simulink model "sixdof"  (R2023a)
settings: Solver=FixedStepAuto  StartTime=0.0  StopTime=5000  FixedStep=0.01  RelTol=1e-3  EnableMultiTasking=on
InitFcn:
  | fox_loadvariables_new
model workspace (MAT data in the model file):
  waypoints = [0 1000 1000 -1000 0 0 0 1000 1000 0 20 20 ... (15 elements, 5x3)]
values from neighbouring files (symbols this model uses):
  Apolar = 0.038    [fox_loadvariables_new.m]
  CD0 = 0.0191    [fox_loadvariables_new.m]
  chord = chord*0.3048    (= 0.3048)    [fox_loadvariables_new.m]
  CL0 = 3*0.076    (= 0.228)    [fox_loadvariables_new.m]
  CLa = 5.097    [fox_loadvariables_new.m]
  CLa_dot = 1.93    [fox_loadvariables_new.m]
  Clb = -0.0598    [fox_loadvariables_new.m]
  ClDa = 0.265    [fox_loadvariables_new.m]
  CLDe = 0.738    [fox_loadvariables_new.m]
  ClDr = 0.0064    [fox_loadvariables_new.m]
  Clp = -0.363    [fox_loadvariables_new.m]
  CLq = 6.03    [fox_loadvariables_new.m]
  Clr = 0.0886    [fox_loadvariables_new.m]
  Cm0 = 0.107    [fox_loadvariables_new.m]
  Cma = -2.051    [fox_loadvariables_new.m]
  Cma_dot = -5.286    [fox_loadvariables_new.m]
  CmDe = -2.021    [fox_loadvariables_new.m]
  Cmq = -16.52    [fox_loadvariables_new.m]
  Cnb = 0.0562    [fox_loadvariables_new.m]
  CnDa = -0.0296    [fox_loadvariables_new.m]
  CnDr = -0.0377    [fox_loadvariables_new.m]
  Cnp = -0.0407    [fox_loadvariables_new.m]
  Cnr = -0.0439    [fox_loadvariables_new.m]
  CYb = -0.204    [fox_loadvariables_new.m]
  CYDr = 0.112    [fox_loadvariables_new.m]
  Euler_0 = [0; 0; 180]'*pi/180    [fox_loadvariables_new.m]
  ISA_g = 9.815    [fox_loadvariables_new.m]
  ISA_hmax = 2000    [fox_loadvariables_new.m]
  ISA_lapse = .0065    (= 0.0065)    [fox_loadvariables_new.m]
  ISA_P0 = 101325    [fox_loadvariables_new.m]
  ISA_R = 287    [fox_loadvariables_new.m]
  ISA_rho0 = 1.225    [fox_loadvariables_new.m]
  ISA_T0 = 289    [fox_loadvariables_new.m]
  Ixx = Ixx*1.355817949    (= 0.363359210332)    [fox_loadvariables_new.m]
  Iyy = Iyy*1.355817949    (= 0.86772348736)    [fox_loadvariables_new.m]
  Izz = Izz*1.355817949    (= 1.19854306692)    [fox_loadvariables_new.m]
  mass = mass*0.45359237    (= 9.0718474)    [fox_loadvariables_new.m]
  Pos_0 = [0; 0; 100.]    [fox_loadvariables_new.m]
  PQR_0 = [0; 0; 0]'    [fox_loadvariables_new.m]
  span = span*0.3048    (= 2.4384)    [fox_loadvariables_new.m]
  Vb_0 = [85.; 0; 0]'*0.3048    [fox_loadvariables_new.m]
undefined symbols (not defined in the file or in its folder): YPGwind
libraries: simulink x5, slpidlib x5, sharedtransform x1, uavutilslib x1, uavalgslib x1
(part 2 of 2)

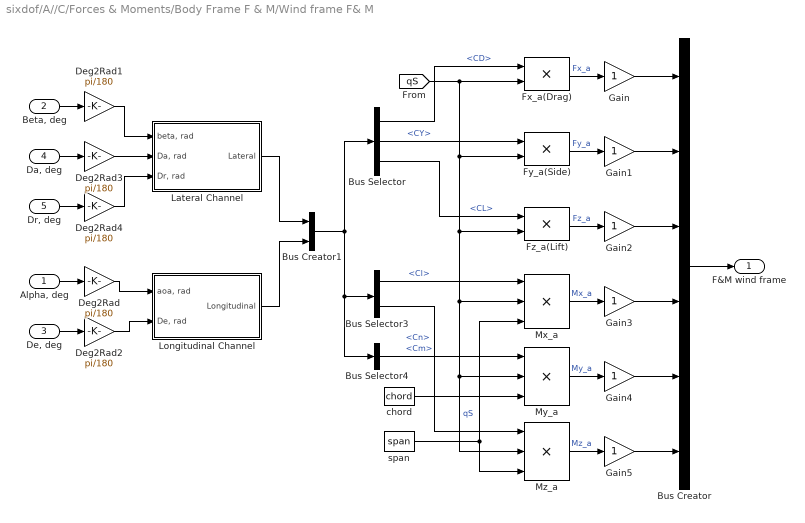
== system sixdof/A//C/Forces & Moments/Body Frame F & M/Wind frame F& M ==
  "Alpha, deg" : Inport
  "Beta, deg" : Inport  Port=2
  "De, deg" : Inport  Port=3
  "Da, deg" : Inport  Port=4
  "Dr, deg" : Inport  Port=5
  Bus Creator : BusCreator  Inputs=6
  Bus Creator1 : BusCreator  Inputs=2
  Bus Selector : BusSelector  OutputSignals=signal2.CD,signal1.CY,signal2.CL
  Bus Selector3 : BusSelector  OutputSignals=signal1.Cl,signal1.Cn
  Bus Selector4 : BusSelector  OutputSignals=signal2.Cm
  Deg2Rad{,1..4} (5 alike) : Gain  Gain=pi/180  SaturateOnIntegerOverflow=on  OutDataTypeStr=Inherit: Same as input  ParamDataTypeStr=Inherit: Same as input
  Fx_a(Drag) : Product  Inputs=**  SaturateOnIntegerOverflow=on  OutDataTypeStr=Inherit: Same as first input
  Fy_a(Side) : Product  SaturateOnIntegerOverflow=on  OutDataTypeStr=Inherit: Same as first input
  Fz_a(Lift) : Product  SaturateOnIntegerOverflow=on  OutDataTypeStr=Inherit: Same as first input
  Gain{,1..5} (6 alike) : Gain  SaturateOnIntegerOverflow=on  OutDataTypeStr=Inherit: Same as input  ParamDataTypeStr=Inherit: Same as input
  Lateral Channel : Subsystem
  Longitudinal Channel : Subsystem
  Mx_a : Product  Inputs=3  SaturateOnIntegerOverflow=on  OutDataTypeStr=Inherit: Same as first input
  My_a : Product  Inputs=3  SaturateOnIntegerOverflow=on  OutDataTypeStr=Inherit: Same as first input
  Mz_a : Product  Inputs=3  SaturateOnIntegerOverflow=on  OutDataTypeStr=Inherit: Same as first input
  chord : Constant  Value=chord  VectorParams1D=off
  span : Constant  Value=span  VectorParams1D=off
  F&M wind frame : Outport
  wires:
  Bus Selector/1 -> Fx_a(Drag)/1  "<CD>"
  Fx_a(Drag)/1 -> Gain/1  "Fx_a"
  Fy_a(Side)/1 -> Gain1/1  "Fy_a"
  Fz_a(Lift)/1 -> Gain2/1  "Fz_a"
  Bus Selector3/1 -> Mx_a/1  "<Cl>"
  Mx_a/1 -> Gain3/1  "Mx_a"
  Bus Selector4/1 -> My_a/1  "<Cm>"
  Mz_a/1 -> Gain5/1  "Mz_a"
  [qS] -> Fx_a(Drag)/2, Fy_a(Side)/2, Fz_a(Lift)/2, Mx_a/2, My_a/2, Mz_a/2  "qS"
  span/1 -> Mx_a/3, Mz_a/3
  chord/1 -> My_a/3
  Bus Selector/2 -> Fy_a(Side)/1  "<CY>"
  Bus Selector/3 -> Fz_a(Lift)/1  "<CL>"
  Bus Selector3/2 -> Mz_a/1  "<Cn>"
  Bus Creator/1 -> F&M wind frame/1
  My_a/1 -> Gain4/1  "My_a"
  Bus Creator1/1 -> Bus Selector/1, Bus Selector3/1, Bus Selector4/1
  Lateral Channel/1(Lateral) -> Bus Creator1/1
  Longitudinal Channel/1(Longitudinal) -> Bus Creator1/2
  "Alpha, deg"/1 -> Deg2Rad/1
  "Beta, deg"/1 -> Deg2Rad1/1
  "De, deg"/1 -> Deg2Rad2/1
  "Da, deg"/1 -> Deg2Rad3/1
  "Dr, deg"/1 -> Deg2Rad4/1
  Deg2Rad1/1 -> Lateral Channel/1("beta, rad")
  Deg2Rad3/1 -> Lateral Channel/2("Da, rad")
  Deg2Rad4/1 -> Lateral Channel/3("Dr, rad")
  Deg2Rad/1 -> Longitudinal Channel/1("aoa, rad")
  Deg2Rad2/1 -> Longitudinal Channel/2("De, rad")
  Gain/1 -> Bus Creator/1
  Gain1/1 -> Bus Creator/2
  Gain2/1 -> Bus Creator/3
  Gain3/1 -> Bus Creator/4
  Gain4/1 -> Bus Creator/5
  Gain5/1 -> Bus Creator/6

== system sixdof/A//C/Forces & Moments/U2B1/Rb2u ==
  phi theta psi : Inport
  11 : Fcn  Expr=cos(u[3])*cos(u[2])
  12 : Fcn  Expr=sin(u[3])*cos(u[2])
  13 : Fcn  Expr=-sin(u[2])
  21 : Fcn  Expr=cos(u[3])*sin(u[2])*sin(u[1])-sin(u[3])*cos(u[1])
  22 : Fcn  Expr=sin(u[3])*sin(u[2])*sin(u[1])+cos(u[3])*cos(u[1])
  23 : Fcn  Expr=cos(u[2])*sin(u[1])
  31 : Fcn  Expr=cos(u[3])*sin(u[2])*cos(u[1])+sin(u[3])*sin(u[1])
  32 : Fcn  Expr=sin(u[3])*sin(u[2])*cos(u[1])-cos(u[3])*sin(u[1])
  33 : Fcn  Expr=cos(u[2])*cos(u[1])
  Mux2 : Mux  Inputs=9
  Reshape : Reshape  OutputDimensionality=Customize  OutputDimensions=[3,3]
  DCM : Outport  InitialOutput=0
  wires:
  Reshape/1 -> DCM/1
  phi theta psi/1 -> 12/1, 13/1, 21/1, 22/1, 23/1, 31/1, 32/1, 33/1, 11/1
  Mux2/1 -> Reshape/1
  11/1 -> Mux2/1
  12/1 -> Mux2/2
  13/1 -> Mux2/3
  21/1 -> Mux2/4
  22/1 -> Mux2/5
  23/1 -> Mux2/6
  31/1 -> Mux2/7
  32/1 -> Mux2/8
  33/1 -> Mux2/9

== system sixdof/A//C/Forces & Moments/U2B2/Rb2u ==
  phi theta psi : Inport
  11 : Fcn  Expr=cos(u[3])*cos(u[2])
  12 : Fcn  Expr=sin(u[3])*cos(u[2])
  13 : Fcn  Expr=-sin(u[2])
  21 : Fcn  Expr=cos(u[3])*sin(u[2])*sin(u[1])-sin(u[3])*cos(u[1])
  22 : Fcn  Expr=sin(u[3])*sin(u[2])*sin(u[1])+cos(u[3])*cos(u[1])
  23 : Fcn  Expr=cos(u[2])*sin(u[1])
  31 : Fcn  Expr=cos(u[3])*sin(u[2])*cos(u[1])+sin(u[3])*sin(u[1])
  32 : Fcn  Expr=sin(u[3])*sin(u[2])*cos(u[1])-cos(u[3])*sin(u[1])
  33 : Fcn  Expr=cos(u[2])*cos(u[1])
  Mux2 : Mux  Inputs=9
  Reshape : Reshape  OutputDimensionality=Customize  OutputDimensions=[3,3]
  DCM : Outport  InitialOutput=0
  wires:
  33/1 -> Mux2/9
  32/1 -> Mux2/8
  31/1 -> Mux2/7
  23/1 -> Mux2/6
  22/1 -> Mux2/5
  21/1 -> Mux2/4
  13/1 -> Mux2/3
  12/1 -> Mux2/2
  11/1 -> Mux2/1
  Mux2/1 -> Reshape/1
  phi theta psi/1 -> 11/1, 33/1, 32/1, 31/1, 23/1, 22/1, 21/1, 13/1, 12/1
  Reshape/1 -> DCM/1

== system sixdof/A//C/ISA Atmosphere & Winds/Wind model/GetWind ==
  Alt : Inport
  "   " : Gain  SaturateOnIntegerOverflow=on  OutDataTypeStr=Inherit: Same as input  ParamDataTypeStr=Inherit: Same as input
  "   1" : Gain  SaturateOnIntegerOverflow=on  OutDataTypeStr=Inherit: Same as input  ParamDataTypeStr=Inherit: Same as input
  "   2" : Gain  SaturateOnIntegerOverflow=on  OutDataTypeStr=Inherit: Same as input  ParamDataTypeStr=Inherit: Same as input
  Mux : Mux  Inputs=3
  WindX : Lookup  InputValues=YPGwind(:,1)  Table=YPGwind(:,3)
  WindY : Lookup  InputValues=YPGwind(:,1)  Table=YPGwind(:,2)
  WindZ : Lookup  InputValues=YPGwind(:,1)  Table=YPGwind(:,4)
  WindOut : Outport  InitialOutput=0
  wires:
  WindY/1 -> "   1"/1
  Alt/1 -> WindZ/1, WindX/1, WindY/1
  WindX/1 -> "   "/1
  "   1"/1 -> Mux/2
  "   "/1 -> Mux/1
  "   2"/1 -> Mux/3
  WindZ/1 -> "   2"/1
  Mux/1 -> WindOut/1

== system sixdof/A//C/Forces & Moments/Body Frame F & M/Transfer to body frame/Ra2b1 ==
  wind frame : Inport
  aoa/beta : Inport  Port=2
  Product2 : Product  Multiplication=Matrix(*)  SaturateOnIntegerOverflow=on  OutDataTypeStr=Inherit: Same as first input
  Ra2b : Math  Operator=transpose  SignedPower=on
  Rb2a : Subsystem
  Reshape : Reshape  OutputDimensionality=Column vector (2-D)
  body frame : Outport
  wires:
  Rb2a/1(Rw2b) -> Ra2b/1
  aoa/beta/1 -> Rb2a/1(aoa beta)
  Product2/1 -> body frame/1
  wind frame/1 -> Reshape/1
  Reshape/1 -> Product2/2
  Ra2b/1 -> Product2/1

== system sixdof/A//C/Forces & Moments/Body Frame F & M/Transfer to body frame/Ra2b22 ==
  aoa/beta : Inport
  wind frame : Inport  Port=2
  Product2 : Product  Multiplication=Matrix(*)  SaturateOnIntegerOverflow=on  OutDataTypeStr=Inherit: Same as first input
  Ra2b : Math  Operator=transpose  SignedPower=on
  Rb2a : Subsystem
  Reshape : Reshape  OutputDimensionality=Column vector (2-D)
  body frame : Outport
  wires:
  Reshape/1 -> Product2/2
  wind frame/1 -> Reshape/1
  Product2/1 -> body frame/1
  aoa/beta/1 -> Rb2a/1(aoa beta)
  Rb2a/1(Rw2b) -> Ra2b/1
  Ra2b/1 -> Product2/1

== system sixdof/A//C/Forces & Moments/Body Frame F & M/Wind frame F& M/Lateral Channel ==
  "beta, rad" : Inport
  "Da, rad" : Inport  Port=2
  "Dr, rad" : Inport  Port=3
  Bus Creator : BusCreator  Inputs=3
  CY : Subsystem
  Cl : Subsystem
  Cn : Subsystem
  Lateral : Outport
  wires:
  Bus Creator/1 -> Lateral/1
  CY/1(CY) -> Bus Creator/1  "CY"
  Cl/1(Cl) -> Bus Creator/2  "Cl"
  Cn/1(Cn) -> Bus Creator/3  "Cn"
  "beta, rad"/1 -> CY/1(beta_dot), Cl/1(beta_dot), Cn/1(beta)
  "Da, rad"/1 -> Cl/2(Da), Cn/2(Da)
  "Dr, rad"/1 -> Cn/3(Dr), Cl/3(Dr), CY/2(Dr)

== system sixdof/A//C/Forces & Moments/Body Frame F & M/Wind frame F& M/Longitudinal Channel ==
  "aoa, rad" : Inport
  "De, rad" : Inport  Port=2
  Bus Creator : BusCreator  Inputs=3
  CD : Subsystem
  CL : Subsystem
  Cm : Subsystem
  Gain : Gain  Gain=-1  SaturateOnIntegerOverflow=on  OutDataTypeStr=Inherit: Same as input  ParamDataTypeStr=Inherit: Same as input
  Gain1 : Gain  Gain=-1  SaturateOnIntegerOverflow=on  OutDataTypeStr=Inherit: Same as input  ParamDataTypeStr=Inherit: Same as input
  Longitudinal : Outport
  wires:
  "aoa, rad"/1 -> Cm/1(alpha), CL/1(alpha)
  CD/1(CD) -> Gain/1
  Gain/1 -> Bus Creator/1  "CD"
  Gain1/1 -> Bus Creator/2  "CL"
  ? -> CL/2(alpha_dot), Cm/2(alpha_dot)
  "De, rad"/1 -> CL/3(De), Cm/3(De)
  CL/1(CL) -> Gain1/1, CD/1(CL)
  Cm/1(Cm) -> Bus Creator/3  "Cm"
  Bus Creator/1 -> Longitudinal/1

== system sixdof/A//C/Forces & Moments/Body Frame F & M/Transfer to body frame/Ra2b1/Rb2a ==
  aoa beta : Inport
  11 : Fcn  Expr=cos(u[1])*cos(u[2])
  12 : Fcn  Expr=sin(u[2])
  13 : Fcn  Expr=sin(u[1])*cos(u[2])
  21 : Fcn  Expr=-cos(u[1])*sin(u[2])
  22 : Fcn  Expr=cos(u[2])
  23 : Fcn  Expr=-sin(u[1])*sin(u[2])
  31 : Fcn  Expr=-sin(u[1])
  32 : Fcn  Expr=0
  33 : Fcn  Expr=cos(u[1])
  Mux3 : Mux  Inputs=9
  Reshape 9x1->3x3 : Reshape  OutputDimensionality=Customize  OutputDimensions=[3,3]
  Rw2b : Outport  InitialOutput=0
  wires:
  aoa beta/1 -> 11/1, 21/1, 31/1, 12/1, 22/1, 32/1, 13/1, 23/1, 33/1
  Mux3/1 -> Reshape 9x1->3x3/1
  Reshape 9x1->3x3/1 -> Rw2b/1
  11/1 -> Mux3/1
  21/1 -> Mux3/2
  31/1 -> Mux3/3
  12/1 -> Mux3/4
  22/1 -> Mux3/5
  32/1 -> Mux3/6
  13/1 -> Mux3/7
  23/1 -> Mux3/8
  33/1 -> Mux3/9

== system sixdof/A//C/Forces & Moments/Body Frame F & M/Transfer to body frame/Ra2b22/Rb2a ==
  aoa beta : Inport
  11 : Fcn  Expr=cos(u[1]) * cos(u[2])
  12 : Fcn  Expr=sin(u[2])
  13 : Fcn  Expr=sin(u[1]) * cos(u[2])
  21 : Fcn  Expr=-cos(u[1]) * sin(u[2])
  22 : Fcn  Expr=cos(u[2])
  23 : Fcn  Expr=-sin(u[1]) * sin(u[2])
  31 : Fcn  Expr=-sin(u[1])
  32 : Fcn  Expr=0
  33 : Fcn  Expr=cos(u[1])
  Mux3 : Mux  Inputs=9
  Reshape 9x1->3x3 : Reshape  OutputDimensionality=Customize  OutputDimensions=[3,3]
  Rw2b : Outport  InitialOutput=0
  wires:
  33/1 -> Mux3/9
  23/1 -> Mux3/8
  13/1 -> Mux3/7
  32/1 -> Mux3/6
  22/1 -> Mux3/5
  12/1 -> Mux3/4
  31/1 -> Mux3/3
  21/1 -> Mux3/2
  11/1 -> Mux3/1
  Reshape 9x1->3x3/1 -> Rw2b/1
  Mux3/1 -> Reshape 9x1->3x3/1
  aoa beta/1 -> 33/1, 23/1, 13/1, 32/1, 22/1, 12/1, 31/1, 21/1, 11/1

== system sixdof/A//C/Forces & Moments/Body Frame F & M/Wind frame F& M/Lateral Channel/CY ==
  beta_dot : Inport
  Dr : Inport  Port=2
  CYDr : Constant  Value=CYDr
  CYb : Constant  Value=CYb
  Gain1 : Gain  SaturateOnIntegerOverflow=on  OutDataTypeStr=Inherit: Same as input  ParamDataTypeStr=Inherit: Same as input
  Gain2 : Gain  SaturateOnIntegerOverflow=on  OutDataTypeStr=Inherit: Same as input  ParamDataTypeStr=Inherit: Same as input
  Product : Product  SaturateOnIntegerOverflow=on  OutDataTypeStr=Inherit: Same as first input
  Product1 : Product  SaturateOnIntegerOverflow=on  OutDataTypeStr=Inherit: Same as first input
  Sum2 : Sum  SaturateOnIntegerOverflow=on
  CY : Outport
  wires:
  CYb/1 -> Product/1
  Product/1 -> Gain1/1
  beta_dot/1 -> Product/2
  Sum2/1 -> CY/1
  Gain1/1 -> Sum2/1
  CYDr/1 -> Product1/1
  Product1/1 -> Gain2/1
  Dr/1 -> Product1/2
  Gain2/1 -> Sum2/2

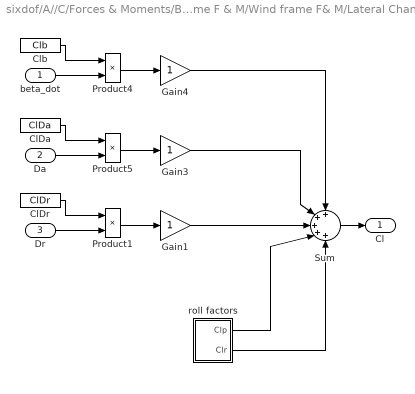
== system sixdof/A//C/Forces & Moments/Body Frame F & M/Wind frame F& M/Lateral Channel/Cl ==
  beta_dot : Inport
  Da : Inport  Port=2
  Dr : Inport  Port=3
  ClDa : Constant  Value=ClDa
  ClDr : Constant  Value=ClDr
  Clb : Constant  Value=Clb
  Gain1 : Gain  SaturateOnIntegerOverflow=on  OutDataTypeStr=Inherit: Same as input  ParamDataTypeStr=Inherit: Same as input
  Gain3 : Gain  SaturateOnIntegerOverflow=on  OutDataTypeStr=Inherit: Same as input  ParamDataTypeStr=Inherit: Same as input
  Gain4 : Gain  SaturateOnIntegerOverflow=on  OutDataTypeStr=Inherit: Same as input  ParamDataTypeStr=Inherit: Same as input
  Product1 : Product  SaturateOnIntegerOverflow=on  OutDataTypeStr=Inherit: Same as first input
  Product4 : Product  SaturateOnIntegerOverflow=on  OutDataTypeStr=Inherit: Same as first input
  Product5 : Product  SaturateOnIntegerOverflow=on  OutDataTypeStr=Inherit: Same as first input
  Sum : Sum  Inputs=+++++  SaturateOnIntegerOverflow=on
  roll factors : Subsystem
  Cl : Outport
  wires:
  Clb/1 -> Product4/1
  Product4/1 -> Gain4/1
  beta_dot/1 -> Product4/2
  ClDa/1 -> Product5/1
  Product5/1 -> Gain3/1
  Da/1 -> Product5/2
  ClDr/1 -> Product1/1
  Product1/1 -> Gain1/1
  Dr/1 -> Product1/2
  Sum/1 -> Cl/1
  Gain4/1 -> Sum/1
  Gain3/1 -> Sum/2
  Gain1/1 -> Sum/3
  roll factors/2(Clr) -> Sum/5
  roll factors/1(Clp) -> Sum/4

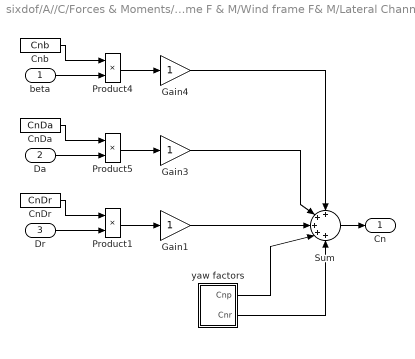
== system sixdof/A//C/Forces & Moments/Body Frame F & M/Wind frame F& M/Lateral Channel/Cn ==
  beta : Inport
  Da : Inport  Port=2
  Dr : Inport  Port=3
  CnDa : Constant  Value=CnDa
  CnDr : Constant  Value=CnDr
  Cnb : Constant  Value=Cnb
  Gain1 : Gain  SaturateOnIntegerOverflow=on  OutDataTypeStr=Inherit: Same as input  ParamDataTypeStr=Inherit: Same as input
  Gain3 : Gain  SaturateOnIntegerOverflow=on  OutDataTypeStr=Inherit: Same as input  ParamDataTypeStr=Inherit: Same as input
  Gain4 : Gain  SaturateOnIntegerOverflow=on  OutDataTypeStr=Inherit: Same as input  ParamDataTypeStr=Inherit: Same as input
  Product1 : Product  SaturateOnIntegerOverflow=on  OutDataTypeStr=Inherit: Same as first input
  Product4 : Product  SaturateOnIntegerOverflow=on  OutDataTypeStr=Inherit: Same as first input
  Product5 : Product  SaturateOnIntegerOverflow=on  OutDataTypeStr=Inherit: Same as first input
  Sum : Sum  Inputs=+++++  SaturateOnIntegerOverflow=on
  yaw factors : Subsystem
  Cn : Outport
  wires:
  yaw factors/1(Cnp) -> Sum/4
  yaw factors/2(Cnr) -> Sum/5
  Gain1/1 -> Sum/3
  Gain3/1 -> Sum/2
  Gain4/1 -> Sum/1
  Sum/1 -> Cn/1
  Dr/1 -> Product1/2
  Product1/1 -> Gain1/1
  CnDr/1 -> Product1/1
  Da/1 -> Product5/2
  Product5/1 -> Gain3/1
  CnDa/1 -> Product5/1
  beta/1 -> Product4/2
  Product4/1 -> Gain4/1
  Cnb/1 -> Product4/1

== system sixdof/A//C/Forces & Moments/Body Frame F & M/Wind frame F& M/Longitudinal Channel/CD ==
  CL : Inport
  Apolar : Constant  Value=Apolar
  CD0 : Constant  Value=CD0
  Product : Product  SaturateOnIntegerOverflow=on  OutDataTypeStr=Inherit: Same as first input
  Product1 : Product  RndMeth=Zero
  Sum1 : Sum  SaturateOnIntegerOverflow=on
  CD : Outport
  wires:
  Sum1/1 -> CD/1
  CD0/1 -> Sum1/1
  Apolar/1 -> Product/1
  Product/1 -> Sum1/2
  CL/1 -> Product1/2, Product1/1
  Product1/1 -> Product/2

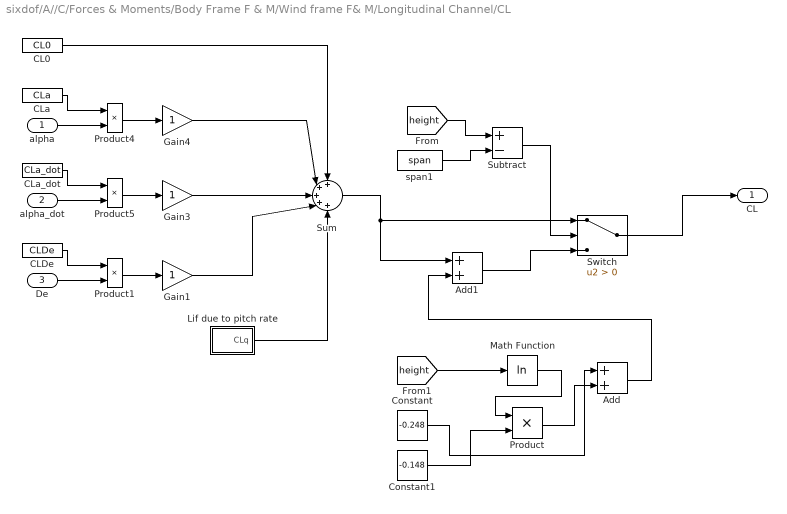
== system sixdof/A//C/Forces & Moments/Body Frame F & M/Wind frame F& M/Longitudinal Channel/CL ==
  alpha : Inport
  alpha_dot : Inport  Port=2
  De : Inport  Port=3
  Add : Sum
  Add1 : Sum
  CL0 : Constant  Value=CL0
  CLDe : Constant  Value=CLDe
  CLa : Constant  Value=CLa
  CLa_dot : Constant  Value=CLa_dot
  Constant : Constant  Value=-0.248
  Constant1 : Constant  Value=-0.148
  Gain1 : Gain  SaturateOnIntegerOverflow=on  OutDataTypeStr=Inherit: Same as input  ParamDataTypeStr=Inherit: Same as input
  Gain3 : Gain  SaturateOnIntegerOverflow=on  OutDataTypeStr=Inherit: Same as input  ParamDataTypeStr=Inherit: Same as input
  Gain4 : Gain  SaturateOnIntegerOverflow=on  OutDataTypeStr=Inherit: Same as input  ParamDataTypeStr=Inherit: Same as input
  Lif due to pitch rate : Subsystem
  Math Function : Math  Operator=log
  Product : Product
  Product1 : Product  SaturateOnIntegerOverflow=on  OutDataTypeStr=Inherit: Same as first input
  Product4 : Product  SaturateOnIntegerOverflow=on  OutDataTypeStr=Inherit: Same as first input
  Product5 : Product  SaturateOnIntegerOverflow=on  OutDataTypeStr=Inherit: Same as first input
  Subtract : Sum  Inputs=+-
  Sum : Sum  Inputs=+++++  SaturateOnIntegerOverflow=on
  Switch : Switch  Criteria=u2 > Threshold  SaturateOnIntegerOverflow=off  InputSameDT=off
  span1 : Constant  Value=span  VectorParams1D=off
  CL : Outport
  wires:
  CLa/1 -> Product4/1
  Product4/1 -> Gain4/1
  alpha/1 -> Product4/2
  CLa_dot/1 -> Product5/1
  Product5/1 -> Gain3/1
  alpha_dot/1 -> Product5/2
  CLDe/1 -> Product1/1
  Product1/1 -> Gain1/1
  De/1 -> Product1/2
  Gain3/1 -> Sum/3
  Gain4/1 -> Sum/2
  CL0/1 -> Sum/1
  Lif due to pitch rate/1(CLq) -> Sum/5
  Gain1/1 -> Sum/4
  Sum/1 -> Add1/1, Switch/1
  [height] -> Subtract/1
  span1/1 -> Subtract/2
  Subtract/1 -> Switch/2
  [height] -> Math Function/1
  Math Function/1 -> Product/1
  Constant1/1 -> Product/2
  Constant/1 -> Add/1
  Product/1 -> Add/2
  Add/1 -> Add1/2
  Add1/1 -> Switch/3
  Switch/1 -> CL/1

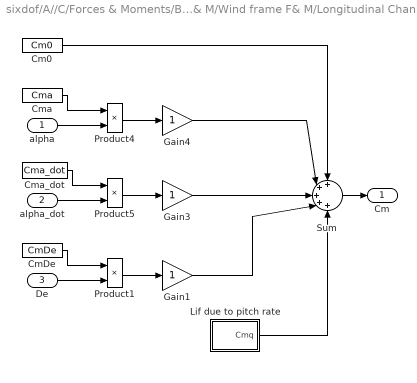
== system sixdof/A//C/Forces & Moments/Body Frame F & M/Wind frame F& M/Longitudinal Channel/Cm ==
  alpha : Inport
  alpha_dot : Inport  Port=2
  De : Inport  Port=3
  Cm0 : Constant  Value=Cm0
  CmDe : Constant  Value=CmDe
  Cma : Constant  Value=Cma
  Cma_dot : Constant  Value=Cma_dot
  Gain1 : Gain  SaturateOnIntegerOverflow=on  OutDataTypeStr=Inherit: Same as input  ParamDataTypeStr=Inherit: Same as input
  Gain3 : Gain  SaturateOnIntegerOverflow=on  OutDataTypeStr=Inherit: Same as input  ParamDataTypeStr=Inherit: Same as input
  Gain4 : Gain  SaturateOnIntegerOverflow=on  OutDataTypeStr=Inherit: Same as input  ParamDataTypeStr=Inherit: Same as input
  Lif due to pitch rate : Subsystem
  Product1 : Product  SaturateOnIntegerOverflow=on  OutDataTypeStr=Inherit: Same as first input
  Product4 : Product  SaturateOnIntegerOverflow=on  OutDataTypeStr=Inherit: Same as first input
  Product5 : Product  SaturateOnIntegerOverflow=on  OutDataTypeStr=Inherit: Same as first input
  Sum : Sum  Inputs=+++++  SaturateOnIntegerOverflow=on
  Cm : Outport
  wires:
  Gain1/1 -> Sum/4
  Lif due to pitch rate/1(Cmq) -> Sum/5
  Cm0/1 -> Sum/1
  Gain4/1 -> Sum/2
  Gain3/1 -> Sum/3
  Sum/1 -> Cm/1
  De/1 -> Product1/2
  Product1/1 -> Gain1/1
  CmDe/1 -> Product1/1
  alpha_dot/1 -> Product5/2
  Product5/1 -> Gain3/1
  Cma_dot/1 -> Product5/1
  alpha/1 -> Product4/2
  Product4/1 -> Gain4/1
  Cma/1 -> Product4/1

== system sixdof/A//C/Forces & Moments/Body Frame F & M/Wind frame F& M/Lateral Channel/Cl/roll factors ==
  Constant : Constant  Value=Clp
  Constant1 : Constant  Value=Clr
  Product : Product  SaturateOnIntegerOverflow=on  OutDataTypeStr=Inherit: Same as first input
  Product1 : Product  SaturateOnIntegerOverflow=on  OutDataTypeStr=Inherit: Same as first input
  Slider Gain : simulink/Math Operations/Slider Gain  gain=1  low=-5  high=5
  Slider Gain1 : simulink/Math Operations/Slider Gain  gain=1  low=-5  high=5
  roll rate fact : Subsystem
  yaw rate fact : Subsystem
  Clp : Outport
  Clr : Outport  Port=2
  wires:
  yaw rate fact/1(Out1) -> Product1/1
  roll rate fact/1(Out1) -> Product/2
  Constant/1 -> Slider Gain/1
  Constant1/1 -> Slider Gain1/1
  Slider Gain1/1 -> Product1/2
  Slider Gain/1 -> Product/1
  Product/1 -> Clp/1
  Product1/1 -> Clr/1

== system sixdof/A//C/Forces & Moments/Body Frame F & M/Wind frame F& M/Lateral Channel/Cn/yaw factors ==
  Constant : Constant  Value=Cnp
  Constant1 : Constant  Value=Cnr
  Product : Product  SaturateOnIntegerOverflow=on  OutDataTypeStr=Inherit: Same as first input
  Product1 : Product  SaturateOnIntegerOverflow=on  OutDataTypeStr=Inherit: Same as first input
  Slider Gain : simulink/Math Operations/Slider Gain  gain=1  low=-5  high=5
  Slider Gain1 : simulink/Math Operations/Slider Gain  gain=1  low=-5  high=5
  roll rate fact : Subsystem
  yaw rate fact : Subsystem
  Cnp : Outport
  Cnr : Outport  Port=2
  wires:
  Product1/1 -> Cnr/1
  Product/1 -> Cnp/1
  Slider Gain/1 -> Product/1
  Slider Gain1/1 -> Product1/2
  Constant1/1 -> Slider Gain1/1
  Constant/1 -> Slider Gain/1
  roll rate fact/1(Out1) -> Product/2
  yaw rate fact/1(Out1) -> Product1/1

== system sixdof/A//C/Forces & Moments/Body Frame F & M/Wind frame F& M/Longitudinal Channel/CL/Lif due to pitch rate ==
  Constant : Constant  Value=CLq
  Product : Product  SaturateOnIntegerOverflow=on  OutDataTypeStr=Inherit: Same as first input
  pitch rate factor : Subsystem
  CLq : Outport
  wires:
  pitch rate factor/1(Out1) -> Product/2
  Constant/1 -> Product/1
  Product/1 -> CLq/1

== system sixdof/A//C/Forces & Moments/Body Frame F & M/Wind frame F& M/Longitudinal Channel/Cm/Lif due to pitch rate ==
  Constant : Constant  Value=Cmq
  Product : Product  SaturateOnIntegerOverflow=on  OutDataTypeStr=Inherit: Same as first input
  Slider Gain : simulink/Math Operations/Slider Gain  gain=1  low=-5  high=5
  pitch rate factor : Subsystem
  Cmq : Outport
  wires:
  Product/1 -> Cmq/1
  Slider Gain/1 -> Product/1
  Constant/1 -> Slider Gain/1
  pitch rate factor/1(Out1) -> Product/2

== system sixdof/A//C/Forces & Moments/Body Frame F & M/Wind frame F& M/Lateral Channel/Cl/roll factors/roll rate fact ==
  Cmq1 : Constant  Value=.5
  Cmq2 : Constant  Value=span
  Product : Product  Inputs=***/  SaturateOnIntegerOverflow=on  OutDataTypeStr=Inherit: Same as first input
  Out1 : Outport
  wires:
  Product/1 -> Out1/1
  [p] -> Product/1
  Cmq1/1 -> Product/2
  Cmq2/1 -> Product/3
  [magV] -> Product/4

== system sixdof/A//C/Forces & Moments/Body Frame F & M/Wind frame F& M/Lateral Channel/Cl/roll factors/yaw rate fact ==
  Cmq1 : Constant  Value=.5
  Cmq2 : Constant  Value=span
  Product : Product  Inputs=***/  SaturateOnIntegerOverflow=on  OutDataTypeStr=Inherit: Same as first input
  Out1 : Outport
  wires:
  [magV] -> Product/4
  Cmq2/1 -> Product/3
  Cmq1/1 -> Product/2
  [r] -> Product/1
  Product/1 -> Out1/1

== system sixdof/A//C/Forces & Moments/Body Frame F & M/Wind frame F& M/Lateral Channel/Cn/yaw factors/roll rate fact ==
  Cmq1 : Constant  Value=.5
  Cmq2 : Constant  Value=span
  Product : Product  Inputs=***/  SaturateOnIntegerOverflow=on  OutDataTypeStr=Inherit: Same as first input
  Out1 : Outport
  wires:
  [magV] -> Product/4
  Cmq2/1 -> Product/3
  Cmq1/1 -> Product/2
  [p] -> Product/1
  Product/1 -> Out1/1

== system sixdof/A//C/Forces & Moments/Body Frame F & M/Wind frame F& M/Lateral Channel/Cn/yaw factors/yaw rate fact ==
  Cmq1 : Constant  Value=.5
  Cmq2 : Constant  Value=span
  Product : Product  Inputs=***/  SaturateOnIntegerOverflow=on  OutDataTypeStr=Inherit: Same as first input
  Out1 : Outport
  wires:
  Product/1 -> Out1/1
  [r] -> Product/1
  Cmq1/1 -> Product/2
  Cmq2/1 -> Product/3
  [magV] -> Product/4

== system sixdof/A//C/Forces & Moments/Body Frame F & M/Wind frame F& M/Longitudinal Channel/CL/Lif due to pitch rate/pitch rate factor ==
  Cmq2 : Constant  Value=chord
  Product : Product  Inputs=**/  SaturateOnIntegerOverflow=on  OutDataTypeStr=Inherit: Same as first input
  Out1 : Outport
  wires:
  Product/1 -> Out1/1
  [q] -> Product/1
  [magV] -> Product/3
  Cmq2/1 -> Product/2

== system sixdof/A//C/Forces & Moments/Body Frame F & M/Wind frame F& M/Longitudinal Channel/Cm/Lif due to pitch rate/pitch rate factor ==
  Cmq2 : Constant  Value=chord
  Product : Product  Inputs=**/  SaturateOnIntegerOverflow=on  OutDataTypeStr=Inherit: Same as first input
  Out1 : Outport
  wires:
  Cmq2/1 -> Product/2
  [magV] -> Product/3
  [q] -> Product/1
  Product/1 -> Out1/1
